simulink subsystem "VS_Camera_Transform_System"  (R2020b)
settings: Solver=VariableStepAuto  StartTime=0.0  StopTime=10.0  RelTol=1e-3
model mask{W_p_C_0=W_T_C_0.t, W_q_C_0=rotm2quat(W_T_C_0.R)', s_star_end=s_star_end, W_T_Cd=W_T_C_desired.double, noise_perc=0, noise_sample_time=0.1}
  mask prompts: noise_sample_time "Noise Sample Time"
settings Model: Creator=marco  LastModifiedBy=marco

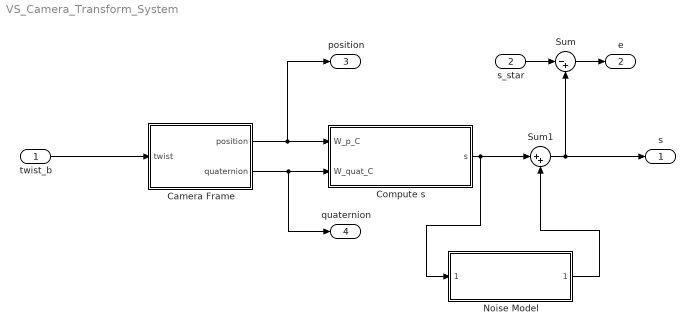
== system VS_Camera_Transform_System ==
  twist_b : Inport
  s_star : Inport  Port=2
  Camera Frame : Subsystem
  Compute s : MATLAB Function  TreatAsAtomicUnit=on
  Noise Model : Subsystem  ReferencedSubsystem=VSNoiseModel  noise_perc=noise_perc  noise_sample_time=Ts
  Sum : Sum  Inputs=|-+
  Sum1 : Sum  Inputs=|++
  s : Outport
  e : Outport  Port=2
  position : Outport  Port=3
  quaternion : Outport  Port=4
  wires:
  Noise Model/1 -> Sum1/2
  Camera Frame/2(quaternion) -> quaternion/1, Compute s/2(W_quat_C)
  Sum1/1 -> Sum/2, s/1
  s_star/1 -> Sum/1
  Sum/1 -> e/1
  Compute s/1(s) -> Noise Model/1, Sum1/1
  Camera Frame/1(position) -> position/1, Compute s/1(W_p_C)
  twist_b/1 -> Camera Frame/1(twist)

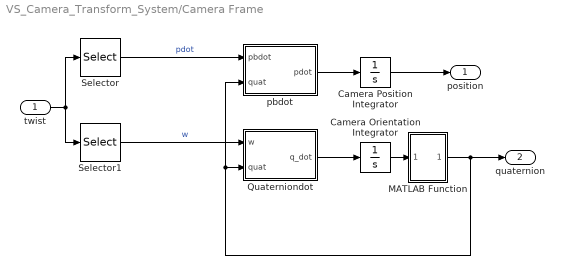
== system VS_Camera_Transform_System/Camera Frame ==
  twist : Inport
  Camera Orientation Integrator : Integrator  InitialCondition=W_q_C_0
  Camera Position Integrator : Integrator  InitialCondition=W_p_C_0
  MATLAB Function : MATLAB Function  TreatAsAtomicUnit=on
  Quaterniondot : MATLAB Function  TreatAsAtomicUnit=on
  Selector : Selector  InputPortWidth=6  IndexOptions=Index vector (dialog)  Indices=[1:3]  OutputSizes=1
  Selector1 : Selector  InputPortWidth=6  IndexOptions=Index vector (dialog)  Indices=[4:6]  OutputSizes=1
  pbdot : MATLAB Function  TreatAsAtomicUnit=on
  position : Outport
  quaternion : Outport  Port=2
  wires:
  twist/1 -> Selector/1, Selector1/1
  Selector/1 -> pbdot/1(pbdot)  "pdot"
  Selector1/1 -> Quaterniondot/1(w)  "w"
  Camera Position Integrator/1 -> position/1
  Quaterniondot/1(q_dot) -> Camera Orientation Integrator/1
  Camera Orientation Integrator/1 -> MATLAB Function/1("quat ")
  pbdot/1(pdot) -> Camera Position Integrator/1
  MATLAB Function/1(quat) -> quaternion/1, pbdot/2(quat), Quaterniondot/2(quat)

== matlab function VS_Camera_Transform_System/Camera Frame/MATLAB Function ==
  data: quat input; quat output
function quat = fcn(quat)

quat = unit(quat);

== matlab function VS_Camera_Transform_System/Camera Frame/Quaterniondot ==
  data: w input; q_dot output; quat input
function q_dot = fcn(w, quat)

q_dot = quat_dotb(quat,w);
% Q = UnitQuaternion(quat);
% Q_dot = Q.dot(w);
% q_dot = Q_dot.double'; 
% q_dot = [0 0 0 0]';

== matlab function VS_Camera_Transform_System/Camera Frame/pbdot ==
  data: pbdot input; pdot output; quat input
function pdot = fcn(pbdot, quat)

W_R_B = quat2rotm(quat');
pdot = W_R_B*pbdot;

== matlab function VS_Camera_Transform_System/Compute s ==
  data: W_p_C input; s output; W_quat_C input; s_star_end parameter; W_T_Cd parameter
function s = fcn(W_p_C, W_quat_C, s_star_end, W_T_Cd)

% W_T_C = SE3(quat2rotm(W_quat_C'),W_p_C);
W_T_C = [quat2rotm(W_quat_C'), W_p_C; 0 0 0 1];

% C_features = inv(W_T_C) * params.W_T_O * params.O_features;
C_T_Cd = invSE3(W_T_C) * W_T_Cd;
C_features = zeros(3,numel(s_star_end)/3);
C_features = homtrans(C_T_Cd, reshape(s_star_end,3,numel(s_star_end)/3));

s = C_features(:);

% s = params.O_features(:);
